simulink model "EVTOLTiltrotor"  (R2024b)
settings: Solver=ode1  StartTime=0.0  StopTime=simTime  RelTol=1e-3  AbsTol=1e-3
undefined symbols (not defined in the file): battery, CityMission, control, FixedWingMission, flightState, FSState, HoverMission, iniRoll, initPitch, iniYaw, params, percWeightGain, position, R_LOOKAHEAD, tiltIni, TransitionMission, uavParam, UAVSampleTime, vIni, Vt, xGround, yGround, zGround
libraries: uavalgslib x7, simulink x4, sharedtransform x2, shared6dof x1, simulink_extras x1, sim3dlib x1, uavsim3dlib x1, uavutilslib x1
(part 2 of 2)

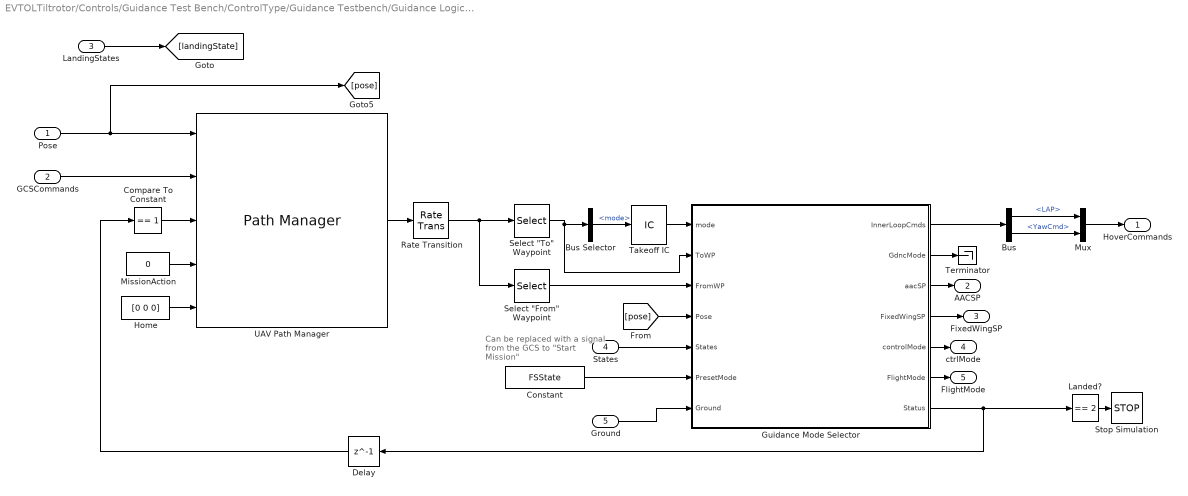
== system EVTOLTiltrotor/Controls/Guidance Test Bench/ControlType/Guidance Testbench/Guidance Logic/Guidance Stateflow ==
  note: Can be replaced with a signal from the GCS to "Start Mission"
  Pose : Inport
  GCSCommands : Inport  Port=2
  LandingStates : Inport  Port=3
  States : Inport  Port=4
  Ground : Inport  Port=5
  "Bus " : BusSelector  OutputSignals=LAP,YawCmd
  Bus Selector : BusSelector  OutputSignals=mode
  Compare To Constant : simulink/Logic and Bit Operations/Compare To Constant  relop===  const=1  OutDataTypeStr=boolean
  Constant : Constant  Value=FSState
  Delay : Delay  DelayLength=1  InitialCondition=0
  Guidance Mode Selector : Stateflow chart  TreatAsAtomicUnit=on  SystemSampleTime=0.02
      settings: PortSchema="{\"entries\":[{\"content\":{\"sides\":[{\"content\":{\"connectorIds\":[\"In1\",\"In2\",\"In3\",\"In4\",\"In5\",\"In6\",\"In7\"]},\"type\":\"ConnectorPlacement.EquallySpacedRectSide\",\"uuid\":\"a9cfd0e2-196c-422d-b359-9161a47768c9\"},{\"content\":{\"connectorIds\":[\"Out7\",\"Out2\",\"Out3\",\"Out4\",\"Out5\",\"Out6\",\"Out1\"],\"side\":\"RIGHT\"},\"type\":\"ConnectorPlacement.EquallySpacedRectSide\",\"uuid\":\"4fed41ae-e7cf-4de3-8bdb-9e24e7d8b079\"},{\"content\":{\"side\":\"TOP\"},\"type\":\"ConnectorPlacement.EquallySpacedRectSide\",\"uuid\":\"2d49ff20-2f63-498d-ac9d-820eae01f794\"}]},\"type\":\"ConnectorPlacement.EquallySpacedConnector\",\"uuid\":\"88d403f4-ad96-40f9-9697-84906f26a8bf\"}],\"packageUris\":[\"http://schema.mathworks.com/mf0/Connector/R2020b\"],\"version\":\"1.0\"}"
  Home : Constant  Value=[0 0 0]  OutDataTypeStr=double
  Landed? : simulink/Logic and Bit Operations/Compare To Constant  relop===  const=2  OutDataTypeStr=boolean
  MissionAction : Constant  Value=0  OutDataTypeStr=uint8
  Mux : Mux  Inputs=2
  Rate Transition : RateTransition
  "Select \"From\" Waypoint" : Selector  InputPortWidth=2  IndexOptions=Index vector (dialog)  Indices=2  OutputSizes=1
  "Select \"To\" Waypoint" : Selector  InputPortWidth=2  IndexOptions=Index vector (dialog)  Indices=1  OutputSizes=1
  Stop Simulation : Stop
  Takeoff IC : InitialCondition
  Terminator : Terminator
  UAV Path Manager : uavalgslib/Path Manager  UAVType=multirotor  LoiterRadius=25  dataType=double  inputBusName='doubleUavPathManager'  SimulateUsing=Code generation
  HoverCommands : Outport
  AACSP : Outport  Port=2
  FixedWingSP : Outport  Port=3
  ctrlMode : Outport  Port=4
  FlightMode : Outport  Port=5
  wires:
  Takeoff IC/1 -> Guidance Mode Selector/1(mode)
  MissionAction/1 -> UAV Path Manager/4
  Guidance Mode Selector/1(Status) -> Delay/1, Landed?/1
  Home/1 -> UAV Path Manager/5
  GCSCommands/1 -> UAV Path Manager/2
  UAV Path Manager/1 -> Rate Transition/1
  Bus Selector/1 -> Takeoff IC/1  "<mode>"
  [pose] -> Guidance Mode Selector/4(Pose)
  Compare To Constant/1 -> UAV Path Manager/3
  "Select \"To\" Waypoint"/1 -> Guidance Mode Selector/2(ToWP), Bus Selector/1
  "Select \"From\" Waypoint"/1 -> Guidance Mode Selector/3(FromWP)
  Landed?/1 -> Stop Simulation/1
  Guidance Mode Selector/2(GdncMode) -> Terminator/1
  Delay/1 -> Compare To Constant/1
  LandingStates/1 -> [landingState]
  States/1 -> Guidance Mode Selector/5(States)
  Guidance Mode Selector/5(controlMode) -> ctrlMode/1
  Guidance Mode Selector/3(aacSP) -> AACSP/1
  Guidance Mode Selector/4(FixedWingSP) -> FixedWingSP/1
  Guidance Mode Selector/6(FlightMode) -> FlightMode/1
  Constant/1 -> Guidance Mode Selector/6(PresetMode)
  "Bus "/1 -> Mux/1  "<LAP>"
  "Bus "/2 -> Mux/2  "<YawCmd>"
  Mux/1 -> HoverCommands/1
  Guidance Mode Selector/7(InnerLoopCmds) -> "Bus "/1
  Ground/1 -> Guidance Mode Selector/7(Ground)
  Pose/1 -> UAV Path Manager/1, [pose]
  Rate Transition/1 -> "Select \"From\" Waypoint"/1, "Select \"To\" Waypoint"/1

== system EVTOLTiltrotor/Controls/Guidance Test Bench/ControlType/Guidance Testbench/Guidance Logic/Interface ==
  UAVState : Inport
  Bus Creator : BusCreator  Inputs=5
  Bus Selector : BusSelector  OutputSignals=Xe,Ve
  Demux : Demux  Outputs=3
  Selector : Selector  InputPortWidth=3  IndexOptions=Index vector (dialog)  Indices=[1]  OutputSizes=1
  Selector1 : Selector  InputPortWidth=3  IndexOptions=Index vector (dialog)  Indices=[2]  OutputSizes=1
  States : Outport
  wires:
  Demux/2 -> Bus Creator/2  "y"
  UAVState/1 -> Bus Selector/1
  Bus Selector/2 -> Selector/1, Selector1/1  "<Ve>"
  Bus Selector/1 -> Demux/1  "<Xe>"
  Demux/1 -> Bus Creator/1  "x"
  Selector/1 -> Bus Creator/4  "vx"
  Demux/3 -> Bus Creator/3  "z"
  Selector1/1 -> Bus Creator/5  "vy"
  Bus Creator/1 -> States/1

== system EVTOLTiltrotor/Controls/Guidance Test Bench/ControlType/Guidance Testbench/Guidance Logic/Subsystem ==
  note: Tilt Angle also determines the state aircraft is in. Thus a unit delay is added
  UAVState : Inport
  Bus Creator : BusCreator  Inputs=6  OutDataTypeStr=Bus: GuidanceStates
  Bus Selector : BusSelector  OutputSignals=Euler,pqr,Ve,Xe,course,RotorParameters.Tilt1
  Gain : Gain
  Unit Delay : UnitDelay  InitialCondition=tiltIni  SampleTime=-1  HasFrameUpgradeWarning=on
  States : Outport
  wires:
  UAVState/1 -> Bus Selector/1
  Bus Selector/1 -> Bus Creator/1  "<Euler>"
  Bus Creator/1 -> States/1
  Bus Selector/3 -> Bus Creator/3  "<Ve>"
  Bus Selector/2 -> Bus Creator/2  "<pqr>"
  Bus Selector/4 -> Bus Creator/4  "<Xe>"
  Bus Selector/5 -> Bus Creator/5  "<course>"
  Gain/1 -> Bus Creator/6  "Tilt"
  Unit Delay/1 -> Gain/1  "Tilt1"
  Bus Selector/6 -> Unit Delay/1  "<Tilt1>"

== system EVTOLTiltrotor/Controls/Guidance Test Bench/ControlType/Manual Control/Command Interface/Control Rate Transition ==
  FM : Inport
  "ControlMode " : Inport  Port=2
  FixedWingSetpoint : Inport  Port=3
  AACSetpoint : Inport  Port=4
  Position : Inport  Port=5
  Rate Transition{,1..3} (4 alike) : RateTransition  OutPortSampleTime=ControlSampleTime
  Rate Transition4 : RateTransition  InitialCondition=flightState.Hover  OutPortSampleTime=ControlSampleTime
  ctrlMode : Outport
  FixedWingSP : Outport  Port=2
  AACSP : Outport  Port=3
  PositionCmds : Outport  Port=4
  FlightMode : Outport  Port=5
  wires:
  Rate Transition4/1 -> FlightMode/1
  Position/1 -> Rate Transition3/1
  FixedWingSetpoint/1 -> Rate Transition1/1
  Rate Transition3/1 -> PositionCmds/1
  FM/1 -> Rate Transition4/1
  "ControlMode "/1 -> Rate Transition/1
  Rate Transition1/1 -> FixedWingSP/1
  AACSetpoint/1 -> Rate Transition2/1
  Rate Transition2/1 -> AACSP/1
  Rate Transition/1 -> ctrlMode/1

== system EVTOLTiltrotor/Controls/Guidance Test Bench/ControlType/Manual Control/Command Interface/Subsystem ==
  note: Tilt Angle also determines the state aircraft is in. Thus a unit delay is added
  UAVState : Inport
  Bus Creator : BusCreator  Inputs=6  OutDataTypeStr=Bus: GuidanceStates
  Bus Selector : BusSelector  OutputSignals=Euler,pqr,Ve,Xe,course,RotorParameters.Tilt1
  Gain : Gain
  Unit Delay : UnitDelay  InitialCondition=tiltIni  SampleTime=-1  HasFrameUpgradeWarning=on
  States : Outport
  wires:
  UAVState/1 -> Bus Selector/1
  Bus Selector/1 -> Bus Creator/1  "<Euler>"
  Bus Creator/1 -> States/1
  Bus Selector/3 -> Bus Creator/3  "<Ve>"
  Bus Selector/2 -> Bus Creator/2  "<pqr>"
  Bus Selector/4 -> Bus Creator/4  "<Xe>"
  Bus Selector/5 -> Bus Creator/5  "<course>"
  Bus Selector/6 -> Unit Delay/1  "<Tilt1>"
  Gain/1 -> Bus Creator/6  "Tilt"
  Unit Delay/1 -> Gain/1  "Tilt2"

== system EVTOLTiltrotor/Controls/Guidance Test Bench/ControlType/Guidance Testbench/Guidance Logic/Guidance Stateflow/Guidance Mode Selector/GuidanceLogic.BackTransition.BackTransition ==
  note: Flight Mode Manager
  States : Inport
  Action Port : ActionPort
      settings: CopyFcn=Stateflow.SLINSF.SimulinkMan.removeBlockPreDeleteFcn  PreDeleteFcn=Stateflow.SLINSF.SimulinkMan.unsafePredeleteFcn
  Bus Creator1 : BusCreator  Inputs=3  OutDataTypeStr=Bus: innerLoopCmdsBus  NonVirtualBus=on
  Bus Selector : BusSelector  OutputSignals=Xe
  Bus Selector1 : BusSelector  OutputSignals=Ve,Tilt
  Constant1 : Constant  Value=0
  Constant2 : Constant  Value=0
  Data Type Conversion : DataTypeConversion  OutDataTypeStr=uint8  SaturateOnIntegerOverflow=off  RndMeth=Floor
  Gain : Gain
  MATLAB Function : MATLAB Function  TreatAsAtomicUnit=on
  Status : Outport
  InnerLoopCmds : Outport  Port=2  OutDataTypeStr=Bus: innerLoopCmdsBus
  wires:
  Bus Selector1/1 -> MATLAB Function/1(Vb)  "<Ve>"
  States/1 -> Bus Selector/1, Bus Selector1/1
  Bus Selector/1 -> Gain/1  "<Xe>"
  Bus Creator1/1 -> InnerLoopCmds/1
  Constant1/1 -> Bus Creator1/2  "HeadingCmd"
  Constant2/1 -> Bus Creator1/3  "YawCmd"
  MATLAB Function/1(flag) -> Data Type Conversion/1
  Data Type Conversion/1 -> Status/1
  Bus Selector1/2 -> MATLAB Function/2(tilt)  "<Tilt>"
  Gain/1 -> Bus Creator1/1  "LAP"

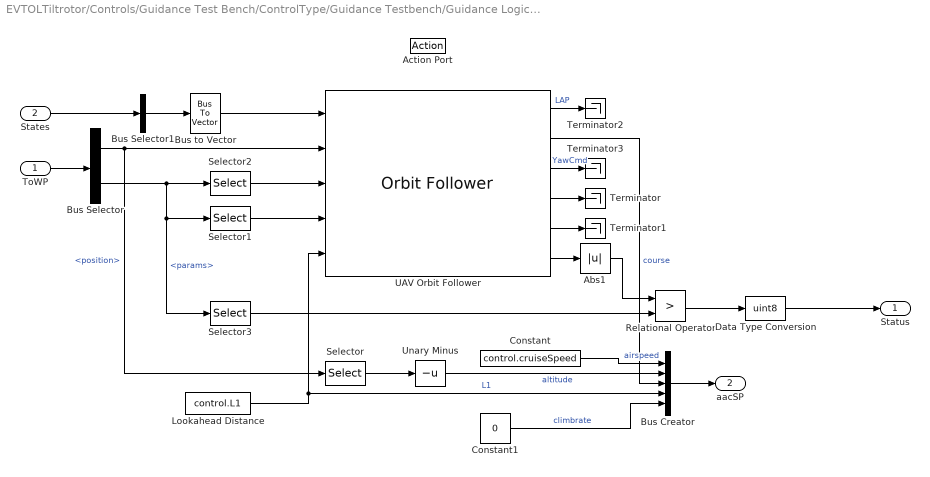
== system EVTOLTiltrotor/Controls/Guidance Test Bench/ControlType/Guidance Testbench/Guidance Logic/Guidance Stateflow/Guidance Mode Selector/GuidanceLogic.FIXED_WING_ORBIT.ORBIT ==
  ToWP : Inport
  States : Inport  Port=2
  Action Port : ActionPort
      settings: CopyFcn=Stateflow.SLINSF.SimulinkMan.removeBlockPreDeleteFcn  PreDeleteFcn=Stateflow.SLINSF.SimulinkMan.unsafePredeleteFcn
  Abs1 : Abs  SaturateOnIntegerOverflow=off
  Bus Creator : BusCreator  Inputs=5  OutDataTypeStr=Bus: AAC  NonVirtualBus=on
      settings: InheritFromInputs=off
  Bus Selector : BusSelector  OutputSignals=position,params
  Bus Selector1 : BusSelector  OutputSignals=Xe,course  OutputAsBus=on
  Bus to Vector : BusToVector
  Constant : Constant  Value=control.cruiseSpeed
  Constant1 : Constant  Value=0
  Data Type Conversion : DataTypeConversion  OutDataTypeStr=uint8  SaturateOnIntegerOverflow=off  RndMeth=Floor
  Lookahead Distance : Constant  Value=control.L1  OutDataTypeStr=double
  Relational Operator : RelationalOperator  Operator=>  OutDataTypeStr=boolean  RndMeth=Simplest  InputSameDT=off
  Selector : Selector  InputPortWidth=3  IndexOptions=Index vector (dialog)  Indices=3  OutputSizes=1
  Selector1 : Selector  InputPortWidth=4  IndexOptions=Index vector (dialog)  Indices=2  OutputSizes=1
  Selector2 : Selector  InputPortWidth=4  IndexOptions=Index vector (dialog)  Indices=1  OutputSizes=1
  Selector3 : Selector  InputPortWidth=4  IndexOptions=Index vector (dialog)  Indices=3  OutputSizes=1
  Terminator{,1..3} (4 alike) : Terminator
  UAV Orbit Follower : uavalgslib/Orbit Follower  UAVType=fixed-wing  MinOrbitRadius=control.turningRadius  MinLookaheadDistance=control.L1  ExternalReset=none  ShowCrossTrackErrorOutput=off  ShowNumTurnsOutput=on  SimulateUsing=Code generation
  Unary Minus : UnaryMinus
  Status : Outport
  aacSP : Outport  Port=2
  wires:
  Bus to Vector/1 -> UAV Orbit Follower/1
  Selector2/1 -> UAV Orbit Follower/3
  Bus Selector/1 -> UAV Orbit Follower/2, Selector/1  "<position>"
  ToWP/1 -> Bus Selector/1
  Bus Selector/2 -> Selector1/1, Selector3/1, Selector2/1  "<params>"
  Selector3/1 -> Relational Operator/2
  Relational Operator/1 -> Data Type Conversion/1
  UAV Orbit Follower/4 -> Terminator/1
  UAV Orbit Follower/5 -> Terminator1/1
  Bus Selector1/1 -> Bus to Vector/1
  States/1 -> Bus Selector1/1
  UAV Orbit Follower/1 -> Terminator2/1  "LAP"
  Lookahead Distance/1 -> UAV Orbit Follower/5, Bus Creator/4  "L1"
  Bus Creator/1 -> aacSP/1
  UAV Orbit Follower/2 -> Bus Creator/3  "course"
  Constant/1 -> Bus Creator/1  "airspeed"
  Unary Minus/1 -> Bus Creator/2  "altitude"
  UAV Orbit Follower/3 -> Terminator3/1  "YawCmd"
  Selector/1 -> Unary Minus/1
  UAV Orbit Follower/6 -> Abs1/1
  Abs1/1 -> Relational Operator/1
  Selector1/1 -> UAV Orbit Follower/4
  Constant1/1 -> Bus Creator/5  "climbrate"
  Data Type Conversion/1 -> Status/1

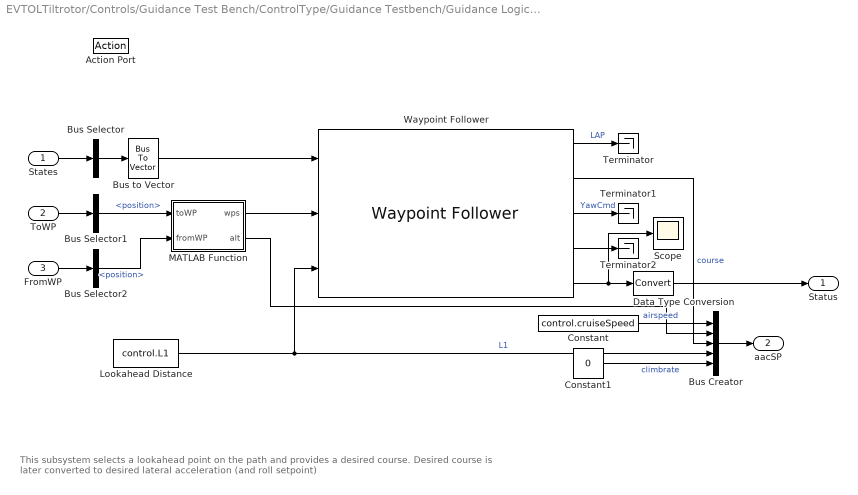
== system EVTOLTiltrotor/Controls/Guidance Test Bench/ControlType/Guidance Testbench/Guidance Logic/Guidance Stateflow/Guidance Mode Selector/GuidanceLogic.FIXED_WING_WAYPOINT.WAYPOINT ==
  note: This subsystem selects a lookahead point on the path and provides a desired course. Desired course is later converted to desired lateral acceleration (and roll setpoint)
  States : Inport
  ToWP : Inport  Port=2
  FromWP : Inport  Port=3
  Action Port : ActionPort
      settings: CopyFcn=Stateflow.SLINSF.SimulinkMan.removeBlockPreDeleteFcn  PreDeleteFcn=Stateflow.SLINSF.SimulinkMan.unsafePredeleteFcn
  Bus Creator : BusCreator  Inputs=5  OutDataTypeStr=Bus: AAC  NonVirtualBus=on
      settings: InheritFromInputs=off
  Bus Selector : BusSelector  OutputSignals=Xe,course  OutputAsBus=on
  Bus Selector1 : BusSelector  OutputSignals=position
  Bus Selector2 : BusSelector  OutputSignals=position
  Bus to Vector : BusToVector
  Constant : Constant  Value=control.cruiseSpeed
  Constant1 : Constant  Value=0
  Data Type Conversion : DataTypeConversion  SaturateOnIntegerOverflow=off  RndMeth=Floor
  Lookahead Distance : Constant  Value=control.L1  OutDataTypeStr=double
  MATLAB Function : MATLAB Function  TreatAsAtomicUnit=on
  Scope : Scope
  Terminator : Terminator
  Terminator1 : Terminator
  Terminator2 : Terminator
  Waypoint Follower : uavalgslib/Waypoint Follower  UAVType=fixed-wing  StartFrom=first  TransitionRadiusSource=internal  TransitionRadius=FWControl.transitionRadius  MinLookaheadDistance=control.L1  HoverAtLastWaypoint=off  YawInput=off  ShowCrossTrackErrorOutput=off  ShowStatusOutput=on  SimulateUsing=Code generation
  Status : Outport
  aacSP : Outport  Port=2
  wires:
  Lookahead Distance/1 -> Waypoint Follower/3, Bus Creator/4  "L1"
  Waypoint Follower/1 -> Terminator/1  "LAP"
  Waypoint Follower/3 -> Terminator1/1  "YawCmd"
  Waypoint Follower/4 -> Terminator2/1
  Constant/1 -> Bus Creator/1  "airspeed"
  States/1 -> Bus Selector/1
  Bus Selector/1 -> Bus to Vector/1
  Waypoint Follower/5 -> Scope/1, Data Type Conversion/1
  Data Type Conversion/1 -> Status/1
  Bus Creator/1 -> aacSP/1
  MATLAB Function/1(wps) -> Waypoint Follower/2
  Bus to Vector/1 -> Waypoint Follower/1
  ToWP/1 -> Bus Selector1/1
  FromWP/1 -> Bus Selector2/1
  Bus Selector1/1 -> MATLAB Function/1(toWP)  "<position>"
  Bus Selector2/1 -> MATLAB Function/2(fromWP)  "<position>"
  MATLAB Function/2(alt) -> Bus Creator/2
  Waypoint Follower/2 -> Bus Creator/3  "course"
  Constant1/1 -> Bus Creator/5  "climbrate"

== system EVTOLTiltrotor/Controls/Guidance Test Bench/ControlType/Guidance Testbench/Guidance Logic/Guidance Stateflow/Guidance Mode Selector/GuidanceLogic.ForwardTransition ==
  Action Port : ActionPort
      settings: CopyFcn=Stateflow.SLINSF.SimulinkMan.removeBlockPreDeleteFcn  PreDeleteFcn=Stateflow.SLINSF.SimulinkMan.unsafePredeleteFcn
  Bus Creator1 : BusCreator  Inputs=3  OutDataTypeStr=Bus: innerLoopCmdsBus  NonVirtualBus=on
  Constant : Constant  Value=0
  Constant1 : Constant  Value=0
  Constant2 : Constant  Value=0
  Constant3 : Constant  Value=[0 0 0]
  Data Type Conversion : DataTypeConversion  OutDataTypeStr=uint8  SaturateOnIntegerOverflow=off  RndMeth=Floor
  Status : Outport
  InnerLoopCmds : Outport  Port=2  OutDataTypeStr=Bus: innerLoopCmdsBus
  wires:
  Constant3/1 -> Bus Creator1/1  "LAP"
  Bus Creator1/1 -> InnerLoopCmds/1
  Constant1/1 -> Bus Creator1/2  "HeadingCmd"
  Constant2/1 -> Bus Creator1/3  "YawCmd"
  Data Type Conversion/1 -> Status/1
  Constant/1 -> Data Type Conversion/1

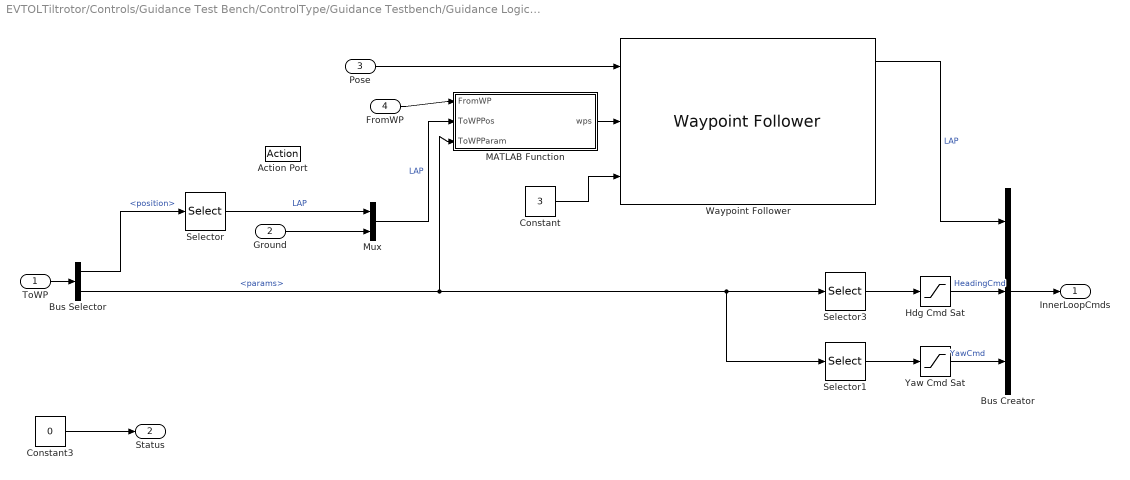
== system EVTOLTiltrotor/Controls/Guidance Test Bench/ControlType/Guidance Testbench/Guidance Logic/Guidance Stateflow/Guidance Mode Selector/GuidanceLogic.Land.Descend ==
  ToWP : Inport
  Ground : Inport  Port=2
  Pose : Inport  Port=3
  FromWP : Inport  Port=4
  Action Port : ActionPort
      settings: CopyFcn=Stateflow.SLINSF.SimulinkMan.removeBlockPreDeleteFcn  PreDeleteFcn=Stateflow.SLINSF.SimulinkMan.unsafePredeleteFcn
  Bus Creator : BusCreator  Inputs=3  OutDataTypeStr=Bus: innerLoopCmdsBus  NonVirtualBus=on
      settings: InheritFromInputs=off
  Bus Selector : BusSelector  OutputSignals=position,params
  Constant : Constant  Value=3
  Constant3 : Constant  Value=0  OutDataTypeStr=uint8
  Hdg Cmd Sat : Saturate  UpperLimit=pi  LowerLimit=-pi
      settings: AttributesFormatString=[%<UpperLimit> %<LowerLimit>]
  MATLAB Function : MATLAB Function  TreatAsAtomicUnit=on
  Mux : Mux  Inputs=2
  Selector : Selector  InputPortWidth=3  IndexOptions=Index vector (dialog)  Indices=[1 2]  OutputSizes=1
  Selector1 : Selector  InputPortWidth=4  IndexOptions=Index vector (dialog)  Indices=4  OutputSizes=1
  Selector3 : Selector  InputPortWidth=4  IndexOptions=Index vector (dialog)  Indices=4  OutputSizes=1
  Waypoint Follower : uavalgslib/Waypoint Follower  UAVType=multirotor  StartFrom=first  TransitionRadiusSource=internal  TransitionRadius=1  MinLookaheadDistance=0.1  HoverAtLastWaypoint=off  YawInput=on  ShowCrossTrackErrorOutput=off  ShowStatusOutput=off  SimulateUsing=Code generation
  Yaw Cmd Sat : Saturate  UpperLimit=pi  LowerLimit=-pi
      settings: AttributesFormatString=[%<UpperLimit> %<LowerLimit>]
  InnerLoopCmds : Outport  OutDataTypeStr=Bus: innerLoopCmdsBus
  Status : Outport  Port=2
  wires:
  Bus Creator/1 -> InnerLoopCmds/1
  Bus Selector/1 -> Selector/1  "<position>"
  Yaw Cmd Sat/1 -> Bus Creator/3  "YawCmd"
  Hdg Cmd Sat/1 -> Bus Creator/2  "HeadingCmd"
  ToWP/1 -> Bus Selector/1
  Selector1/1 -> Yaw Cmd Sat/1
  Selector3/1 -> Hdg Cmd Sat/1
  Selector/1 -> Mux/1  "LAP"
  Bus Selector/2 -> MATLAB Function/3(ToWPParam), Selector1/1, Selector3/1  "<params>"
  Ground/1 -> Mux/2
  Constant3/1 -> Status/1
  Mux/1 -> MATLAB Function/2(ToWPPos)  "LAP"
  FromWP/1 -> MATLAB Function/1(FromWP)
  Pose/1 -> Waypoint Follower/1
  MATLAB Function/1(wps) -> Waypoint Follower/2
  Constant/1 -> Waypoint Follower/3
  Waypoint Follower/1 -> Bus Creator/1  "LAP"

== system EVTOLTiltrotor/Controls/Guidance Test Bench/ControlType/Guidance Testbench/Guidance Logic/Guidance Stateflow/Guidance Mode Selector/GuidanceLogic.Land.ToLand ==
  Pose : Inport
  ToWP : Inport  Port=2
  FromWP : Inport  Port=3
  Action Port : ActionPort
      settings: CopyFcn=Stateflow.SLINSF.SimulinkMan.removeBlockPreDeleteFcn  PreDeleteFcn=Stateflow.SLINSF.SimulinkMan.unsafePredeleteFcn
  Bus Creator1 : BusCreator  Inputs=3  OutDataTypeStr=Bus: innerLoopCmdsBus  NonVirtualBus=on
  Constant : Constant  Value=0  OutDataTypeStr=uint8
  Lookahead Distance : Constant  Value=3  OutDataTypeStr=double
  MATLAB Function : MATLAB Function  TreatAsAtomicUnit=on
  Scope : Scope
  Waypoint Follower : uavalgslib/Waypoint Follower  UAVType=multirotor  StartFrom=first  TransitionRadiusSource=internal  TransitionRadius=1  MinLookaheadDistance=0.1  HoverAtLastWaypoint=off  YawInput=on  ShowCrossTrackErrorOutput=off  ShowStatusOutput=off  SimulateUsing=Code generation
  Status : Outport
  InnerLoopCmds : Outport  Port=2  OutDataTypeStr=Bus: innerLoopCmdsBus
  wires:
  Constant/1 -> Status/1
  MATLAB Function/1(wps) -> Waypoint Follower/2
  Lookahead Distance/1 -> Waypoint Follower/3
  Bus Creator1/1 -> InnerLoopCmds/1
  ToWP/1 -> MATLAB Function/2(ToWP)
  Waypoint Follower/2 -> Bus Creator1/2  "HeadingCmd"
  FromWP/1 -> MATLAB Function/1(FromWP)
  Waypoint Follower/4 -> Scope/1
  Pose/1 -> Waypoint Follower/1
  Waypoint Follower/1 -> Bus Creator1/1  "LAP"
  Waypoint Follower/3 -> Bus Creator1/3  "YawCmd"

== system EVTOLTiltrotor/Controls/Guidance Test Bench/ControlType/Guidance Testbench/Guidance Logic/Guidance Stateflow/Guidance Mode Selector/GuidanceLogic.Orbit ==
  ToWP : Inport
  Pose : Inport  Port=2
  Action Port : ActionPort
      settings: CopyFcn=Stateflow.SLINSF.SimulinkMan.removeBlockPreDeleteFcn  PreDeleteFcn=Stateflow.SLINSF.SimulinkMan.unsafePredeleteFcn
  Abs : Abs  SaturateOnIntegerOverflow=off
  Bus Creator : BusCreator  Inputs=3  OutDataTypeStr=Bus: innerLoopCmdsBus  NonVirtualBus=on
  Bus Selector : BusSelector  OutputSignals=position,params
  Data Type Conversion : DataTypeConversion  OutDataTypeStr=uint8  SaturateOnIntegerOverflow=off  RndMeth=Floor
  Lookahead Distance : Constant  Value=5  OutDataTypeStr=double
  Radius : Selector  InputPortWidth=4  IndexOptions=Index vector (dialog)  Indices=[3]  OutputSizes=1
  Relational Operator : RelationalOperator  Operator=>  OutDataTypeStr=boolean  RndMeth=Simplest  InputSameDT=off
  Sign : Signum  ZeroCross=off
  Terminator : Terminator
  Terminator1 : Terminator
  Turns : Selector  InputPortWidth=4  IndexOptions=Index vector (dialog)  Indices=[1]  OutputSizes=1
  UAV Orbit Follower : uavalgslib/Orbit Follower  UAVType=multirotor  MinOrbitRadius=1  MinLookaheadDistance=0.1  ExternalReset=none  ShowCrossTrackErrorOutput=off  ShowNumTurnsOutput=on  SimulateUsing=Code generation
  InnerLoopCmds : Outport  OutDataTypeStr=Bus: innerLoopCmdsBus
  Status : Outport  Port=2
  wires:
  Pose/1 -> UAV Orbit Follower/1
  Lookahead Distance/1 -> UAV Orbit Follower/5
  Abs/1 -> UAV Orbit Follower/3
  Bus Selector/1 -> UAV Orbit Follower/2  "<position>"
  ToWP/1 -> Bus Selector/1
  UAV Orbit Follower/1 -> Bus Creator/1  "LAP"
  Bus Creator/1 -> InnerLoopCmds/1
  UAV Orbit Follower/2 -> Bus Creator/2  "HeadingCmd"
  UAV Orbit Follower/3 -> Bus Creator/3  "YawCmd"
  Bus Selector/2 -> Turns/1, Radius/1  "<params>"
  Radius/1 -> Abs/1, Sign/1
  Sign/1 -> UAV Orbit Follower/4
  Relational Operator/1 -> Data Type Conversion/1
  Turns/1 -> Relational Operator/2
  Data Type Conversion/1 -> Status/1
  UAV Orbit Follower/6 -> Relational Operator/1
  UAV Orbit Follower/4 -> Terminator/1
  UAV Orbit Follower/5 -> Terminator1/1

== system EVTOLTiltrotor/Controls/Guidance Test Bench/ControlType/Guidance Testbench/Guidance Logic/Guidance Stateflow/Guidance Mode Selector/GuidanceLogic.Takeoff ==
  ToWP : Inport
  Pose : Inport  Port=2
  Action Port : ActionPort
      settings: CopyFcn=Stateflow.SLINSF.SimulinkMan.removeBlockPreDeleteFcn  PreDeleteFcn=Stateflow.SLINSF.SimulinkMan.unsafePredeleteFcn
  Bus Creator : BusCreator  Inputs=3  OutDataTypeStr=Bus: innerLoopCmdsBus  NonVirtualBus=on
      settings: InheritFromInputs=off
  Bus Selector : BusSelector  OutputSignals=position,params
  Constant : Constant  Value=0  OutDataTypeStr=uint8
  Constant1 : Constant  Value=0
  Demux : Demux  Outputs=[2 2]
  Demux1 : Demux  Outputs=[2 1]
  Hdg. Cmd Sat : Saturate  UpperLimit=pi  LowerLimit=-pi
      settings: AttributesFormatString=[%<UpperLimit> %<LowerLimit>]
  Mux : Mux  Inputs=2
  Selector3 : Selector  InputPortWidth=4  IndexOptions=Index vector (dialog)  Indices=4  OutputSizes=1
  Terminator : Terminator
  Terminator1 : Terminator
  Yaw Cmd Sat : Saturate  UpperLimit=pi  LowerLimit=-pi
      settings: AttributesFormatString=[%<UpperLimit> %<LowerLimit>]
  InnerLoopCmds : Outport  OutDataTypeStr=Bus: innerLoopCmdsBus
  Status : Outport  Port=2
  wires:
  Hdg. Cmd Sat/1 -> Bus Creator/2  "HeadingCmd"
  Bus Creator/1 -> InnerLoopCmds/1
  Constant/1 -> Status/1
  Pose/1 -> Demux/1
  Yaw Cmd Sat/1 -> Bus Creator/3  "YawCmd"
  ToWP/1 -> Bus Selector/1
  Bus Selector/2 -> Selector3/1  "<params>"
  Mux/1 -> Bus Creator/1  "LAP"
  Demux/1 -> Mux/1
  Bus Selector/1 -> Demux1/1  "<position>"
  Demux/2 -> Terminator/1
  Demux1/1 -> Terminator1/1
  Selector3/1 -> Hdg. Cmd Sat/1
  Constant1/1 -> Yaw Cmd Sat/1
  Demux1/2 -> Mux/2

== system EVTOLTiltrotor/Controls/Guidance Test Bench/ControlType/Guidance Testbench/Guidance Logic/Guidance Stateflow/Guidance Mode Selector/GuidanceLogic.WP ==
  FromWP : Inport
  Pose : Inport  Port=2
  ToWP : Inport  Port=3
  Action Port : ActionPort
      settings: CopyFcn=Stateflow.SLINSF.SimulinkMan.removeBlockPreDeleteFcn  PreDeleteFcn=Stateflow.SLINSF.SimulinkMan.unsafePredeleteFcn
  Back Transition Guard : Subsystem
  Bus Creator : BusCreator  Inputs=3  OutDataTypeStr=Bus: innerLoopCmdsBus  NonVirtualBus=on
  Constant : Constant  Value=0
  Data Type Conversion : DataTypeConversion  OutDataTypeStr=uint8  SaturateOnIntegerOverflow=off  RndMeth=Floor
  Dist2WP : Subsystem
  Lookahead Distance : Constant  Value=R_LOOKAHEAD  OutDataTypeStr=double
  MATLAB Function : MATLAB Function  TreatAsAtomicUnit=on
  Relational Operator : RelationalOperator  OutDataTypeStr=boolean  RndMeth=Simplest  InputSameDT=off
  Scope : Scope
  Terminator : Terminator
  Waypoint Follower : uavalgslib/Waypoint Follower  UAVType=multirotor  StartFrom=closest  TransitionRadiusSource=internal  TransitionRadius=R_WAYPOINTTRANSITION  MinLookaheadDistance=0.1  HoverAtLastWaypoint=off  YawInput=on  ShowCrossTrackErrorOutput=off  ShowStatusOutput=off  SimulateUsing=Code generation
  InnerLoopCmds : Outport  OutDataTypeStr=Bus: innerLoopCmdsBus
  Status : Outport  Port=2
  wires:
  Data Type Conversion/1 -> Status/1
  Bus Creator/1 -> InnerLoopCmds/1
  ToWP/1 -> Dist2WP/3(ToWP), MATLAB Function/2(ToWP)
  Waypoint Follower/1 -> Bus Creator/1  "LAP"
  MATLAB Function/1(wps) -> Waypoint Follower/2
  Waypoint Follower/2 -> Bus Creator/2  "HeadingCmd"
  Waypoint Follower/4 -> Scope/1
  Dist2WP/1(Dist) -> Relational Operator/2
  FromWP/1 -> Back Transition Guard/2(FromWP)
  Relational Operator/1 -> Data Type Conversion/1
  Back Transition Guard/1(PrevWP) -> Dist2WP/2(FromWP), MATLAB Function/1(FromWP)
  Pose/1 -> Back Transition Guard/1(Poses), Waypoint Follower/1, Dist2WP/1(Pose)
  Lookahead Distance/1 -> Relational Operator/1, Waypoint Follower/3
  Constant/1 -> Bus Creator/3  "YawCmd"
  Waypoint Follower/3 -> Terminator/1  "YawCmd"

== system EVTOLTiltrotor/Controls/Guidance Test Bench/ControlType/Guidance Testbench/Guidance Logic/Guidance Stateflow/Guidance Mode Selector/GuidanceLogic.WP/Back Transition Guard ==
  note: Set previous waypoint to current location if the UAV has just exited back transition
  Poses : Inport
  FromWP : Inport  Port=2
  Bus Selector : BusSelector  OutputSignals=mode
  Bus Selector1 : BusSelector  OutputSignals=position,params,mode
  Constant : Constant  Value=6
  Equal : RelationalOperator  Operator===  OutDataTypeStr=boolean  RndMeth=Simplest  InputSameDT=off
  Switch : Switch  Criteria=u2 > Threshold  SaturateOnIntegerOverflow=off  InputSameDT=off
  Triggered Subsystem : Subsystem  TreatAsAtomicUnit=on
  Out Bus Element2 : Outport  PortName=PrevWP  Element=mode
  Out Bus Element : Outport  PortName=PrevWP  Element=position
  Out Bus Element1 : Outport  PortName=PrevWP  Element=params
  wires:
  FromWP/1 -> Bus Selector1/1, Bus Selector/1
  Bus Selector/1 -> Equal/2  "<mode>"
  Constant/1 -> Equal/1
  Equal/1 -> Switch/2, Triggered Subsystem/Trigger
  Poses/1 -> Triggered Subsystem/1(Poses)
  Triggered Subsystem/1(HoldPositionValue) -> Switch/1
  Bus Selector1/1 -> Switch/3  "<position>"
  Switch/1 -> Out Bus Element/1
  Bus Selector1/2 -> Out Bus Element1/1  "<params>"
  Bus Selector1/3 -> Out Bus Element2/1  "<mode>"

== system EVTOLTiltrotor/Controls/Guidance Test Bench/ControlType/Guidance Testbench/Guidance Logic/Guidance Stateflow/Guidance Mode Selector/GuidanceLogic.WP/Dist2WP ==
  Pose : Inport
  FromWP : Inport  Port=2
  ToWP : Inport  Port=3
  Bus Selector : BusSelector  OutputSignals=position
  Bus Selector1 : BusSelector  OutputSignals=position
  Demux : Demux  Outputs=[3 1]
  Dot Product : DotProduct  OutDataTypeStr=Inherit: Inherit via internal rule
  Subsystem : Subsystem
  Sum : Sum  Inputs=|-+
  Sum1 : Sum  Inputs=|+-
  Terminator : Terminator
  Dist : Outport
  wires:
  Sum1/1 -> Subsystem/1(V)
  Demux/2 -> Terminator/1
  Bus Selector/1 -> Sum/2, Sum1/1  "<position>"
  Demux/1 -> Sum/1
  Bus Selector1/1 -> Sum1/2  "<position>"
  Sum/1 -> Dot Product/1
  Subsystem/1(V_unit) -> Dot Product/2
  Pose/1 -> Demux/1
  Dot Product/1 -> Dist/1
  ToWP/1 -> Bus Selector/1
  FromWP/1 -> Bus Selector1/1

== system EVTOLTiltrotor/Controls/Guidance Test Bench/ControlType/Guidance Testbench/Guidance Logic/Guidance Stateflow/Guidance Mode Selector/GuidanceLogic.WP/Back Transition Guard/Triggered Subsystem ==
  Poses : Inport
  Trigger : TriggerPort  VariantControl=(inherit)
  Reshape : Reshape  OutputDimensionality=Customize  OutputDimensions=[3,1]
  Selector : Selector  InputPortWidth=4  IndexOptions=Index vector (dialog)  Indices=[1 2 3]  OutputSizes=1
  HoldPositionValue : Outport
  wires:
  Poses/1 -> Selector/1
  Selector/1 -> Reshape/1
  Reshape/1 -> HoldPositionValue/1

== system EVTOLTiltrotor/Controls/Guidance Test Bench/ControlType/Guidance Testbench/Guidance Logic/Guidance Stateflow/Guidance Mode Selector/GuidanceLogic.WP/Dist2WP/Subsystem ==
  V : Inport
  Dot Product1 : DotProduct  OutDataTypeStr=Inherit: Inherit via internal rule
  Product : Product  Inputs=*/
  Saturation : Saturate  UpperLimit=inf  LowerLimit=0.00001
  Sqrt : Sqrt
  V_unit : Outport
  wires:
  V/1 -> Dot Product1/2, Dot Product1/1, Product/1
  Sqrt/1 -> Product/2
  Dot Product1/1 -> Saturation/1
  Saturation/1 -> Sqrt/1
  Product/1 -> V_unit/1

== matlab function EVTOLTiltrotor/Airframe/Ground Truth Bus/Ground Track ==
  data: vxyz input; course output; gndSpeed output
function [course, gndSpeed] = fcn(vxyz)
% Compute the course of the aircrafta and
% ground speed of the aircraft
vx = vxyz(1);
vy = vxyz(2);
course = atan2(vy, vx);
gndSpeed = norm([vx vy 0]);

== matlab function EVTOLTiltrotor/Controls/Sensor/No Sensors Dynamics/MATLAB Function ==
  data: euler input; ypr output
function ypr = fcn(euler)

ypr = [euler(3),euler(2),euler(1)];
end

== stateflow chart EVTOLTiltrotor/Controls/Guidance Test Bench/ControlType/Guidance Testbench/Guidance Logic/Guidance Stateflow/Guidance Mode Selector ==
  settings: updateMethod=DISCRETE  sampleTime=UAVSampleTime*4
  state GuidanceLogic
    state FIXED_WING_WAYPOINT
      en:
      controlMode.airspeedAltitude = 1;
      controlMode.attitude = 1;
      controlMode.lateralGuidance = 1;
      state WAYPOINT
    state FIXED_WING_ENTRY
      state Stabilize
        en:
        FlightMode=flightState.FixedWing;
        controlMode.attitude = 1;
        controlMode.airspeedAltitude = 0;
        controlMode.lateralGuidance = 0;
        %Transition once done.
        FixedWingSP.yaw = 0;
        FixedWingSP.pitch = 0;
        FixedWingSP.roll = 0;
        FixedWingSP.airspeed=15;
        Status= uint8(0);
      state FIXEDWINGFLIGHT
        en:
        % Control mode
        controlMode.airspeedAltitude = 1;
        controlMode.attitude = 1;
        controlMode.lateralGuidance = 1;
        % Setpoint init
        aacSP.L1 = 25;
        aacSP.airspeed = 15;
        aacSP.altitude = 0;
        aacSP.course=0;
      (default) -> Stabilize
      Stabilize -> FIXEDWINGFLIGHT : after(3,sec)
    state Start
      en:
      %Set Flight mode to hover
      FlightMode=PresetMode;
      %Set default settings
      % Control mode
      controlMode.airspeedAltitude = 0;
      controlMode.attitude = 0;
      controlMode.lateralGuidance = 0;
      controlMode.TransitionCondition = 0;
      % Setpoint init
      FixedWingSP.yaw = 0;
      FixedWingSP.pitch = 0;
      FixedWingSP.roll = 0;
      FixedWingSP.airspeed=15;
      aacSP.L1 = 25;
      aacSP.airspeed = 15;
      aacSP.altitude = 0;
      aacSP.course=0;
      InnerLoopCmds.YawCmd=0;
    state FIXED_WING_ORBIT
      en:
      controlMode.airspeedAltitude = 1;
      controlMode.attitude = 1;
      controlMode.lateralGuidance = 1;
      state ORBIT
    state HOVER_ENTRY
      en:
      FlightMode=flightState.Hover;
      controlMode.inTransition=0;
    state Takeoff
    state WP
    state Orbit
    state PreTransition
      en:
      FlightMode=flightState.FixedWing;
      controlMode.airspeedAltitude = 1;
      controlMode.attitude = 1;
      controlMode.lateralGuidance = 1;
      % Setpoint init
      aacSP.L1 = 25;
      aacSP.airspeed = 14;
      aacSP.altitude = altitudeHold;
      aacSP.course=courseHold;
    state BackTransition
      state BackTransition
    state ForwardTransition
    state FWCOMPLETE
      Status=uint8(1);
      controlMode.TransitionCondition=uint8(1);
    note: [(mode==4)]
    state Land
      state Descend
      state ToLand
      (default) -> ToLand
      ToLand -> Descend : [(norm(Pose(1:2)-ToWP.position(1:2)) <= 3)]
    (default) -> Start
    Start -> (junction 5)
    FIXEDWINGFLIGHT -> WAYPOINT [order 2] : [(mode==2)]
        | {Status=uint8(0);}
    FIXEDWINGFLIGHT -> ORBIT [order 1] : [(mode==3)]
        | {Status= uint8(0);}
    (junction 262) -> FIXED_WING_ENTRY
    (junction 5) -> FIXED_WING_ORBIT [order 6] : [(mode==3)&&(FlightMode==flightState.FixedWing)]
        | {Status=uint8(0);}
    (junction 5) -> (junction 262) [order 3] : [(FlightMode==flightState.Transition)]
        | {controlMode.inTransition=0;}
    (junction 255) -> HOVER_ENTRY
    (junction 5) -> (junction 255) [order 4] : [(FlightMode==flightState.BackTransition)]
        | {controlMode.inTransition=0;}
    HOVER_ENTRY -> (junction 12)
    (junction 257) -> FIXED_WING_WAYPOINT
    Takeoff -> WP : [Pose(3) <= ToWP.position(3)]{Status = uint8(1);}
    GuidanceLogic -> (junction 5) : [(hasChanged(mode))]
    (junction 5) -> Takeoff [order 5] : [(mode == 1)&&(FlightMode==flightState.Hover)]
        | {controlMode.inTransition=0;}
    (junction 5) -> (junction 257) [order 2] : [(mode==2)&&(FlightMode==flightState.FixedWing)]
        | {Status=uint8(0);}
    (junction 5) -> (junction 260) [order 1] : [(mode==6)&&(FlightMode==flightState.FixedWing)]
        | {courseHold=States.course;
        | altitudeHold=-States.Xe(3); }
    (junction 5) -> (junction 12) [order 7] : [FlightMode==flightState.Hover]
        | {controlMode.inTransition=0;}
    (junction 260) -> PreTransition
    (junction 12) -> WP [order 1] : [(mode==2)]
    (junction 12) -> (junction 17) [order 2]
    (junction 17) -> Orbit [order 1] : [(mode==3)]
    (junction 17) -> (junction 22) [order 2]
    PreTransition -> GuidanceLogic.BackTransition : after(5,sec)
        | {FlightMode=flightState.BackTransition;
        | controlMode.inTransition=1; }
    (junction 22) -> ForwardTransition [order 1] : [(mode==6)]
        | {FlightMode=flightState.Transition;
        | controlMode.inTransition=1;
        | controlMode.TransitionCondition=uint8(0);
        |
        | }
    (junction 22) -> Land [order 2]
    ForwardTransition -> FWCOMPLETE : [transitionConditionMet(States,Vt)]
  (default) -> GuidanceLogic
  data: sf_internal_action_state_placeholder_data local double size=1 =0; sf_internal_action_state_placeholder_data local double size=1 =0; sf_internal_action_state_placeholder_data local double size=1 =0; sf_internal_action_state_placeholder_data local double size=1 =0; sf_internal_action_state_placeholder_data local double size=1 =0; sf_internal_action_state_placeholder_data local double size=1 =0; sf_internal_action_state_placeholder_data local double size=1 =0; sf_internal_action_state_placeholder_data local double size=1 =0; sf_internal_action_state_placeholder_data local double size=1 =0; TransitionSt function_input Bus: GuidanceStates; valid function_output; Vtransition function_input; mode input; ToWP input Bus: doubleUavPathManager; Status output uint8; FromWP input Bus: doubleUavPathManager; Pose input; GdncMode output Enum: GdncModeType; States input; aacSP output Bus: AAC; FixedWingSP output Bus: FixedWingCommandBus; controlMode output Bus: controlMode; FlightMode output; PresetMode input; courseHold local; altitudeHold local; Vt parameter double; InnerLoopCmds output Bus: innerLoopCmdsBus; zGround parameter; Ground input
  function valid=transitionConditionMet(TransitionSt,Vtransition):
    | function valid=transitionConditionMet(TransitionSt,Vtransition)
    | %wingsLevel
    | if(States.Tilt>=1.57)&&(vecnorm(States.Ve)>Vt)
    |    valid=true;
    | else
    |     valid=false;
    | end
    | end

== matlab function EVTOLTiltrotor/Controls/Guidance Test Bench/ControlType/Guidance Testbench/Guidance Logic/Guidance Stateflow/Guidance Mode Selector/GuidanceLogic.BackTransition.BackTransition/MATLAB Function ==
  data: Vb input; tilt input; flag output
function flag = fcn(Vb,tilt)
tiltConditionMet=abs(tilt)<1e-1;
velocityConditionMet=abs(norm([Vb(1) 0 0]))<4;

flag=tiltConditionMet&velocityConditionMet;
end

== matlab function EVTOLTiltrotor/Controls/Guidance Test Bench/ControlType/Guidance Testbench/Guidance Logic/Guidance Stateflow/Guidance Mode Selector/GuidanceLogic.FIXED_WING_WAYPOINT.WAYPOINT/MATLAB Function ==
  data: toWP input; wps output; fromWP input; alt output
function [wps, alt]= fcn(toWP, fromWP)
    wps = zeros(2,3); %#ok<PREALL> 
    wps = [fromWP'; toWP'];
    alt = -toWP(3);
end

== matlab function EVTOLTiltrotor/Controls/Guidance Test Bench/ControlType/Guidance Testbench/Guidance Logic/Guidance Stateflow/Guidance Mode Selector/GuidanceLogic.Land.Descend/MATLAB Function ==
  data: FromWP input Bus: doubleUavPathManager size=1; wps output; ToWPPos input size=[3 1]; ToWPParam input size=[4 1]
function wps = getLandingWaypoint(FromWP, ToWPPos, ToWPParam)

persistent outWPS

if isempty(outWPS)
    outWPS = double(zeros(2,4));
end

outWPS(1,:) = [FromWP.position' FromWP.params(4)];
outWPS(2,:) = [reshape(ToWPPos,1,[]), ToWPParam(4)];

wps = outWPS;

== matlab function EVTOLTiltrotor/Controls/Guidance Test Bench/ControlType/Guidance Testbench/Guidance Logic/Guidance Stateflow/Guidance Mode Selector/GuidanceLogic.Land.ToLand/MATLAB Function ==
  data: FromWP input Bus: doubleUavPathManager size=1; wps output; ToWP input Bus: doubleUavPathManager size=1
function wps = getLandingWaypoint(FromWP, ToWP)

persistent outWPS

if isempty(outWPS)
    outWPS = double(zeros(2,4));
end

outWPS(1,:) = [FromWP.position' FromWP.params(4)];
outWPS(2,:) = [ToWP.position(1:2)' FromWP.position(3) ToWP.params(4)];

wps = outWPS;

== matlab function EVTOLTiltrotor/Controls/Guidance Test Bench/ControlType/Guidance Testbench/Guidance Logic/Guidance Stateflow/Guidance Mode Selector/GuidanceLogic.WP/MATLAB Function ==
  data: FromWP input Bus: doubleUavPathManager size=1; wps output; ToWP input Bus: doubleUavPathManager size=1
function wps = getWaypointMission(FromWP, ToWP)

persistent outWPS

if isempty(outWPS)
    outWPS = double(zeros(2,4));
end

outWPS(1,:) = [FromWP.position' FromWP.params(4)];
outWPS(2,:) = [ToWP.position' ToWP.params(4)];

wps = outWPS;

== stateflow chart EVTOLTiltrotor/Controls/Guidance Test Bench/ControlType/Manual Control/Command Interface/Basic Control  Switching ==
  state STATE_MACHINE
    state DEFAULT
      en:
      controlMode.lateralGuidance=1;
      controlMode.airspeedAltitude=1;
      controlMode.attitude=1;
      controlMode.manual=0;
      controlMode.armed=0;
      controlMode.inTransition=0;
    state TRANSITION
      controlMode.lateralGuidance=1;
      controlMode.airspeedAltitude=1;
      controlMode.attitude=1;
      controlMode.manual=0;
      controlMode.armed=0;
      controlMode.inTransition=1;
      controlMode.TransitionCondition=0;
    (default) -> DEFAULT
    STATE_MACHINE -> DEFAULT [order 2] : [hasChanged(FlightMode)]
    STATE_MACHINE -> TRANSITION [order 1] : [hasChanged(FlightMode)&&((FlightMode==flightState.Transition)||(FlightMode==flightState.BackTransition))]
    TRANSITION -> STATE_MACHINE [order 2] : [backConditioMet(States)&&(FlightMode==flightState.BackTransition)]
        | {controlMode.TransitionCondition=1;
        | controlMode.inTransition=0;}
    TRANSITION -> STATE_MACHINE [order 1] : [transitionConditionMet(States,Vt)&&(FlightMode==flightState.Transition)]
        | {controlMode.TransitionCondition=1;
        | controlMode.inTransition=0;}
  data: TransitionStates function_input Bus: GuidanceStates; valid function_output; Vtransition function_input; TransitionStates function_input Bus: GuidanceStates; valid function_output; controlMode output Bus: controlMode; FlightMode input; States input; Vt parameter double
  function valid=transitionConditionMet(TransitionStates,Vtransition):
    | function valid=transitionConditionMet(TransitionStates,Vtransition)
    | %wingsLevel
    | if((States.Tilt>=1.57)&&(vecnorm(States.Ve)>Vt))
    |    valid=true;
    | else
    |     valid=false;
    | end
    | end
  function valid=backConditioMet(TransitionStates):
    | function valid=backConditioMet(TransitionStates)
    | %wingsLevel
    | if(vecnorm(States.Ve)<1e-1)
    |    valid=true;
    | else
    |     valid=false;
    | end
    | end
